simulink model "normalFilter"  (R2020a)
settings: Solver=VariableStepAuto  StartTime=0.0  StopTime=tStop  MaxStep=dt  RelTol=1e-3
values from neighbouring files (symbols this model uses):
  noiseAmp = 1    [defaultSignal.m]
  noiseFreq = 50    [defaultSignal.m]
  signalAmp = 10    [defaultSignal.m]
  signalFreq = 1    [defaultSignal.m]
settings Model: Creator=DELL  LastModifiedBy=DELL

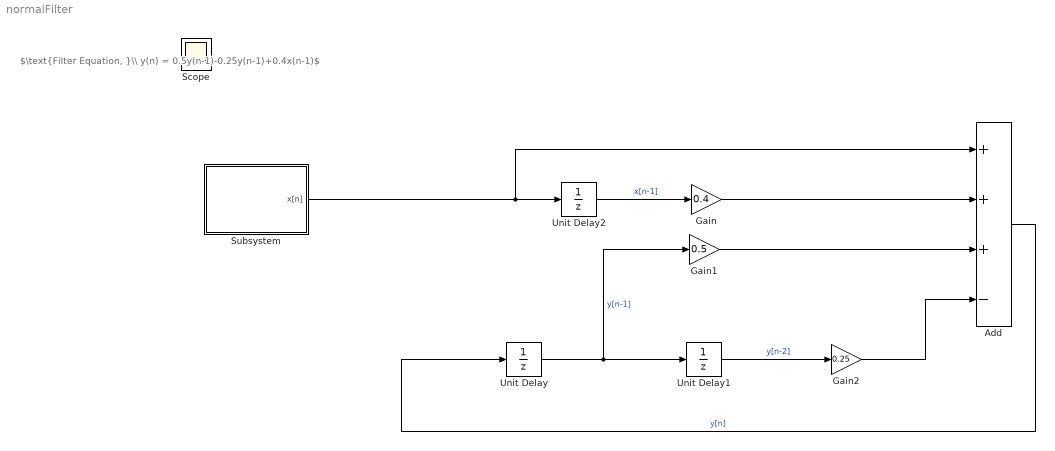
== system normalFilter ==
  note: $\text{Filter Equation, }\\ y(n) = 0.5y(n-1)-0.25y(n-1)+0.4x(n-1)$
  Add : Sum  Inputs=+++-
  Gain : Gain  Gain=0.4
  Gain1 : Gain  Gain=0.5
  Gain2 : Gain  Gain=0.25
  Subsystem : Subsystem
  Unit Delay : UnitDelay  SampleTime=-1  HasFrameUpgradeWarning=on
  Unit Delay1 : UnitDelay  SampleTime=-1  HasFrameUpgradeWarning=on
  Unit Delay2 : UnitDelay  SampleTime=-1  HasFrameUpgradeWarning=on
  Scope : Scope
  wires:
  Add/1 -> Unit Delay/1  "y[n]"
  Unit Delay/1 -> Gain1/1, Unit Delay1/1  "y[n-1]"
  Unit Delay1/1 -> Gain2/1  "y[n-2]"
  Unit Delay2/1 -> Gain/1  "x[n-1]"
  Gain2/1 -> Add/4
  Gain1/1 -> Add/3
  Gain/1 -> Add/2
  Subsystem/1(x[n]) -> Add/1, Unit Delay2/1

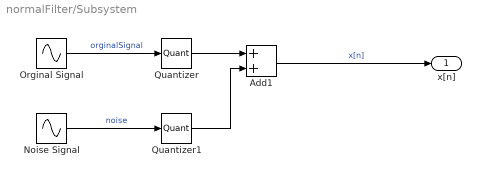
== system normalFilter/Subsystem ==
  Add1 : Sum
  Noise Signal : Sin  Amplitude=noiseAmp  Frequency=2*pi*noiseFreq  SampleTime=0
  Orginal Signal : Sin  Amplitude=signalAmp  Frequency=2*pi*signalFreq  SampleTime=0
  Quantizer : Quantizer
  Quantizer1 : Quantizer
  x[n] : Outport
  wires:
  Orginal Signal/1 -> Quantizer/1  "orginalSignal"
  Add1/1 -> x[n]/1  "x[n]"
  Quantizer1/1 -> Add1/2
  Noise Signal/1 -> Quantizer1/1  "noise"
  Quantizer/1 -> Add1/1
